simulink model "EREV_1_Model_RL"  (R2025a)
settings: Solver=ode4  StartTime=0.0  StopTime=2474  FixedStep=0.05  MaxStep=0.01  RelTol=1e-3
values from neighbouring files (symbols this model uses):
  Af = 2.95    [EREV_RL_Parameters.m]
  bsfc_map = [ ... (first row only)    [EREV_RL_Parameters.m]
  Cd = 0.33    [EREV_RL_Parameters.m]
  eff_map_F = [ ... (first row only)    [EREV_RL_Parameters.m]
  eff_map_R = [ ... (first row only)    [EREV_RL_Parameters.m]
  eff_spd_F_rpm = [0    1000  2000  3000  4000  5000  6000  7000  8000  9000  10000 11000 12000]    [EREV_RL_Parameters.m]
  eff_spd_R_rpm = [0    1000  2000  3000  4000  5000  6000  7000  8000  9000  10000 11000 12000 13000 14000 15000]    [EREV_RL_Parameters.m]
  eff_trq_F = [0   26   53   79   106  132  158  185  211  238  264]    [EREV_RL_Parameters.m]
  eff_trq_R = [0   30   61   91   122  152  182  213  243  274  304]    [EREV_RL_Parameters.m]
  eng_speed_bsfc = [1000  1500  2000  2500  3000  3500  4000  4500  5000]    [EREV_RL_Parameters.m]
  eng_speed_rpm = [1000  1500  2000  2500  3000  3500  4000  4500  5000  5500  6000]    [EREV_RL_Parameters.m]
  eng_sweet_spot_speed = 2200    [EREV_RL_Parameters.m]
  eng_sweet_spot_torque = 180    [EREV_RL_Parameters.m]
  eng_torque_bsfc = [0  50  100  150  200  250]    [EREV_RL_Parameters.m]
  eng_torque_curve = [180   240   265   265   255   240   220   195   170   145   120]    [EREV_RL_Parameters.m]
  f_roll = 0.008    [EREV_RL_Parameters.m]
  g = 9.81    [EREV_RL_Parameters.m]
  G_final_F = 8.0    (= 8)    [EREV_RL_Parameters.m]
  G_final_R_1st = G_1st    (= 12)    [EREV_RL_Parameters.m]
  G_final_R_2nd = G_2nd    (= 7)    [EREV_RL_Parameters.m]
  h = 0.65    [EREV_RL_Parameters.m]
  M_veh = 2165    [EREV_RL_Parameters.m]
  Q_bat_Ah = 38.3    [EREV_RL_Parameters.m]
  Q_bat_kWh = 13.8    [EREV_RL_Parameters.m]
  R_int_base = 0.15    [EREV_RL_Parameters.m]
  R_multiplier = [3.0  2.0  1.5  1.2  1.1  1.0  1.0  1.1  1.2  1.8  2.5]    [EREV_RL_Parameters.m]
  r_tire = 0.369    [EREV_RL_Parameters.m]
  rho = 1.225    [EREV_RL_Parameters.m]
  shift_duration = 0.3    [EREV_RL_Parameters.m]
  SOC_init = 0.5    [EREV_RL_Parameters.m]
  SOC_R_table = [0.0  0.1  0.2  0.3  0.4  0.5  0.6  0.7  0.8  0.9  1.0]    [EREV_RL_Parameters.m]
  T_motor_F_curve = [264  264  264   264   264   250   230   210   195   180   168                      156  145   135   126   118   111   104    98    92    87    82    77    73    68]    [EREV_RL_Parameters.m]
  T_motor_R_curve = [304  304  304   304   304   304   295   280   265   250   235                      220  205   192   180   169   159   150   141   133   126   119                      113  107   101    96    91    86    82    78    74]    [EREV_RL_Parameters.m]
  T_motor_R_max = 304    [EREV_RL_Parameters.m]
  T_wheel_brake_max = 5000    [EREV_RL_Parameters.m]
  tau_m_F = 0.02    [EREV_RL_Parameters.m]
  tau_m_R = 0.02    [EREV_RL_Parameters.m]
  theta = 0    [EREV_RL_Parameters.m]
  torque_split_F_4wd = 0.4    [EREV_RL_Parameters.m]
  torque_split_R_4wd = 0.6    [EREV_RL_Parameters.m]
  V_downshift_kph = 30    [EREV_RL_Parameters.m]
  v_regen_min = 8    [EREV_RL_Parameters.m]
  V_upshift_kph = 35    [EREV_RL_Parameters.m]
  VOC_map = No_cell * VOC_cell    [EREV_RL_Parameters.m]
  VOC_SOC = [0    0.05  0.1   0.2   0.3   0.4   0.5   0.6   0.7   0.8   0.9   0.95  1.0]    [EREV_RL_Parameters.m]
  Vt_init = 374.4    [EREV_RL_Parameters.m]
  w_motor_F_rpm = [0    500  1000  1500  2000  2500  3000  3500  4000  4500  5000                    5500  6000  6500  7000  7500  8000  8500  9000  9500  10000 10500 11000 11500 12000]    [EREV_RL_Parameters.m]
  w_motor_R_rpm = [0    500  1000  1500  2000  2500  3000  3500  4000  4500  5000                    5500  6000  6500  7000  7500  8000  8500  9000  9500  10000 10500                   11000 11500 12000 12500 13000 13500 14000 14500 15000]    [EREV_RL_Parameters.m]
undefined symbols (not defined in the file or in its folder): T_brake_max, T_wheel_max_current
libraries: simulink x2, autolibshared x1, slpidlib x1, rllib x1
(part 1 of 2)
settings Model: SimulationMode=accelerator  Creator=wnsgu  LastModifiedBy=wnsgu
settings SolverCC: ZeroCrossAlgorithm=Adaptive
settings DataIOCC: DSMLogging=off  ReturnWorkspaceOutputs=off

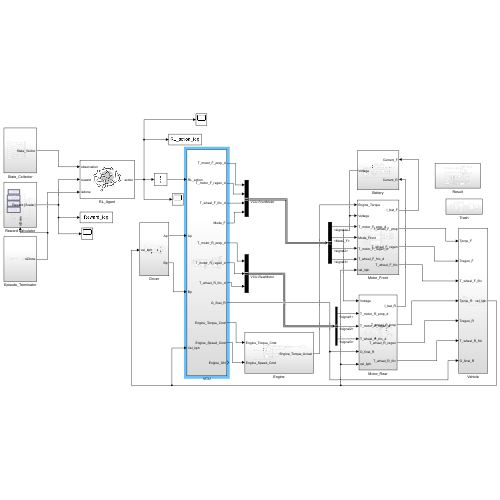
[thumbnail: Simulink's stored preview of the top-level diagram]
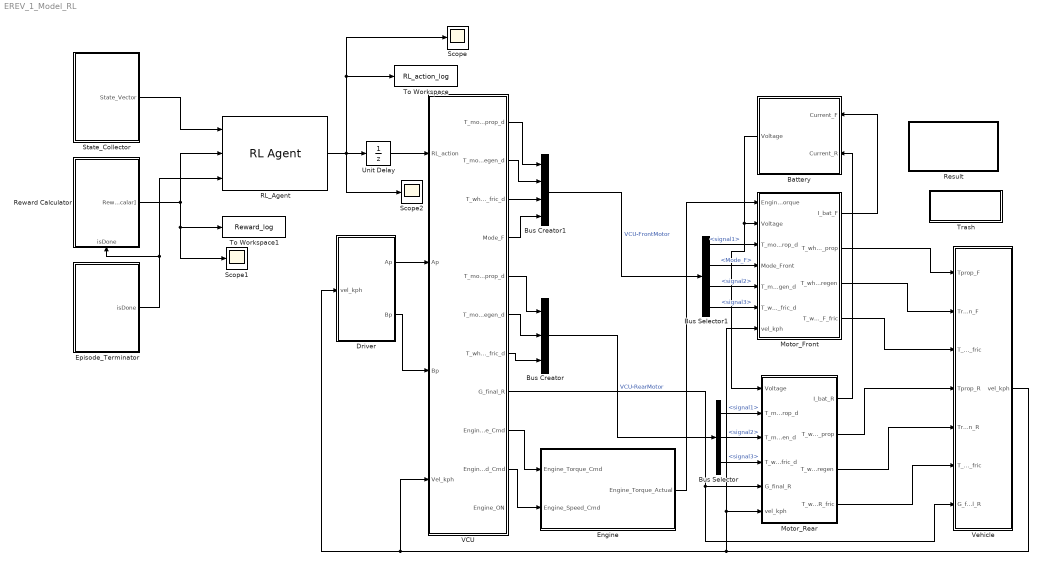
== system EREV_1_Model_RL ==
  Battery : Subsystem
      settings: PortSchema="{\"entries\":[{\"content\":{\"sides\":[{\"content\":{},\"type\":\"ConnectorPlacement.EquallySpacedRectSide\",\"uuid\":\"439f0e77-8416-4342-b481-750735cf5ce5\"},{\"content\":{\"side\":\"RIGHT\"},\"type\":\"ConnectorPlacement.EquallySpacedRectSide\",\"uuid\":\"9523e7eb-47b9-4e0c-8038-141b83390da7\"},{\"content\":{\"connectorIds\":[\"In1\",\"In2\"],\"side\":\"TOP\"},\"type\":\"ConnectorPlacement.EquallySpacedRectSide\",\"uuid\":\"5c1be694-faa9-41f0-8cd7-b694ba64a7e5\"},{\"content\":{\"connectorIds\":[\"Out1\"],\"side\":\"BOTTOM\"},\"type\":\"ConnectorPlacement.EquallySpacedRectSide\",\"uuid\":\"71711254-1c62-4381-9e1d-0f8c6cd96e13\"}]},\"type\":\"ConnectorPlacement.EquallySpacedConnector\",\"uuid\":\"675be46a-f4a3-46ab-8639-2a4821ad0461\"}],\"packageUris\":[\"http://schema.mathworks.com/mf0/Connector/R2020b\"],\"version\":\"1.0\"}"
  Bus Creator : BusCreator  Inputs=3
  Bus Creator1 : BusCreator  Inputs=4
  Bus Selector : BusSelector  OutputSignals=signal1,signal2,signal3
  Bus Selector1 : BusSelector  OutputSignals=signal1,Mode_F,signal2,signal3
  Driver : Subsystem
  Engine : Subsystem
      settings: PortSchema="{\"entries\":[{\"content\":{\"sides\":[{\"content\":{\"connectorIds\":[\"Out1\"]},\"type\":\"ConnectorPlacement.EquallySpacedRectSide\",\"uuid\":\"b19a6c52-e995-4cc1-a102-0e3cd4878d2e\"},{\"content\":{\"connectorIds\":[\"In1\",\"In2\"],\"side\":\"RIGHT\"},\"type\":\"ConnectorPlacement.EquallySpacedRectSide\",\"uuid\":\"94e23d2a-046b-4832-bf19-f0caf19abac1\"},{\"content\":{\"side\":\"TOP\"},\"type\":\"ConnectorPlacement.EquallySpacedRectSide\",\"uuid\":\"5633464f-1f19-4555-82ba-daafa5aadce4\"}]},\"type\":\"ConnectorPlacement.EquallySpacedConnector\",\"uuid\":\"3cf45f49-ebfb-4ab6-bab2-429e9c87361e\"}],\"packageUris\":[\"http://schema.mathworks.com/mf0/Connector/R2020b\"],\"version\":\"1.0\"}"
  Episode_Terminator : Subsystem
  Motor_Front : Subsystem
  Motor_Rear : Subsystem
  RL_Agent : rllib/RL Agent  Agent=agent  ExternalActionAsInput=off  ProvideLastAction=off  ProvideCumRwd=off  TreatAsDirectFeedthrough=on  UseStrictObservationDataTypes=off
  Result : Subsystem
  Reward Calculator : Subsystem
      settings: PortSchema="{\"entries\":[{\"content\":{\"sides\":[{\"content\":{},\"type\":\"ConnectorPlacement.EquallySpacedRectSide\",\"uuid\":\"cfaed86a-057d-4c04-868d-776f7886e6b3\"},{\"content\":{\"connectorIds\":[\"Out1\"],\"side\":\"RIGHT\"},\"type\":\"ConnectorPlacement.EquallySpacedRectSide\",\"uuid\":\"d11a40b4-e160-4fac-ae26-3ae90e992ab0\"},{\"content\":{\"side\":\"TOP\"},\"type\":\"ConnectorPlacement.EquallySpacedRectSide\",\"uuid\":\"52ab05fd-eff5-43dc-9a3c-d65837210fcf\"},{\"content\":{\"connectorIds\":[\"In1\"],\"side\":\"BOTTOM\"},\"type\":\"ConnectorPlacement.EquallySpacedRectSide\",\"uuid\":\"e3afb124-135f-4d45-89ab-9c20129580e4\"}]},\"type\":\"ConnectorPlacement.EquallySpacedConnector\",\"uuid\":\"1111a298-f3ef-4593-8227-a04b6f8dfe1f\"}],\"packageUris\":[\"http://schema.mathworks.com/mf0/Connector/R2020b\"],\"version\":\"1.0\"}"
  Scope : Scope
      settings: ActiveDisplayYMinimum=1  ActiveDisplayYMaximum=3  DataLoggingVariableName=ScopeData20
  Scope1 : Scope
      settings: ActiveDisplayYMinimum=-0.0074059355050510745  ActiveDisplayYMaximum=0.0037360945819499259  DataLoggingVariableName=ScopeData19
  Scope2 : Scope
      settings: ActiveDisplayYMinimum=-1  ActiveDisplayYMaximum=1  DataLoggingVariableName=ScopeData2
  State_Collector : Subsystem
  To Workspace : ToWorkspace  VariableName=RL_action_log  SaveFormat=Timeseries  SampleTime=-1
  To Workspace1 : ToWorkspace  VariableName=Reward_log  SaveFormat=Timeseries  SampleTime=-1
  Trash : Subsystem
  Unit Delay : UnitDelay  SampleTime=-1  HasFrameUpgradeWarning=on
  VCU : Subsystem
  Vehicle : Subsystem
  wires:
  Driver/2(Bp) -> VCU/3(Bp)
  Vehicle/1(vel_kph) -> VCU/4(Vel_kph), Driver/1(vel_kph), Motor_Rear/6(vel_kph), Motor_Front/7(vel_kph)
  Driver/1(Ap) -> VCU/2(Ap)
  VCU/9(Engine_Torque_Cmd) -> Engine/2(Engine_Torque_Cmd)
  VCU/10(Engine_Speed_Cmd) -> Engine/1(Engine_Speed_Cmd)
  Engine/1(Engine_Torque_Actual) -> Motor_Front/1(Engine_Torque)
  Motor_Front/2(T_wheel_F_prop) -> Vehicle/1(Tprop_F)
  Motor_Front/3(T_wheel_F_regen) -> Vehicle/2(Tregen_F)
  Motor_Front/4(T_wheel_F_fric) -> Vehicle/3(T_wheel_F_fric)
  Battery/1(Voltage) -> Motor_Rear/1(Voltage), Motor_Front/2(Voltage)
  Motor_Rear/1(I_bat_R) -> Battery/2(Current_R)
  Motor_Front/1(I_bat_F) -> Battery/1(Current_F)
  Motor_Rear/2(T_wheel_R_prop) -> Vehicle/4(Tprop_R)
  Motor_Rear/3(T_wheel_R_regen) -> Vehicle/5(Tregen_R)
  Motor_Rear/4(T_wheel_R_fric) -> Vehicle/6(T_wheel_R_fric)
  VCU/8(G_final_R) -> Motor_Rear/5(G_final_R), Vehicle/7(G_final_R)
  VCU/5(T_motor_R_prop_d) -> Bus Creator/1
  VCU/6(T_motor_R_regen_d) -> Bus Creator/2
  VCU/7(T_wheel_R_fric_d) -> Bus Creator/3
  Bus Creator/1 -> Bus Selector/1  "VCU-RearMotor"
  Bus Selector/2 -> Motor_Rear/3(T_motor_R_regen_d)  "<signal2>"
  Bus Selector/1 -> Motor_Rear/2(T_motor_R_prop_d)  "<signal1>"
  Bus Selector/3 -> Motor_Rear/4(T_wheel_R_fric_d)  "<signal3>"
  VCU/4(Mode_F) -> Bus Creator1/4
  Bus Creator1/1 -> Bus Selector1/1  "VCU-FrontMotor"
  VCU/1(T_motor_F_prop_d) -> Bus Creator1/1
  VCU/2(T_motor_F_regen_d) -> Bus Creator1/2
  VCU/3(T_wheel_F_fric_d) -> Bus Creator1/3
  Bus Selector1/1 -> Motor_Front/3(T_motor_F_prop_d)  "<signal1>"
  Bus Selector1/4 -> Motor_Front/6(T_wheel_F_fric_d)  "<signal3>"
  Reward Calculator/1(Reward [Scalar]) -> RL_Agent/2, Scope1/1, To Workspace1/1
  RL_Agent/1 -> Scope/1, To Workspace/1, Scope2/1, Unit Delay/1
  State_Collector/1(State_Vector) -> RL_Agent/1
  Episode_Terminator/1(isDone) -> RL_Agent/3, Reward Calculator/1(isDone)
  Bus Selector1/2 -> Motor_Front/4(Mode_Front)  "<Mode_F>"
  Bus Selector1/3 -> Motor_Front/5(T_motor_F_regen_d)  "<signal2>"
  Unit Delay/1 -> VCU/1(RL_action)

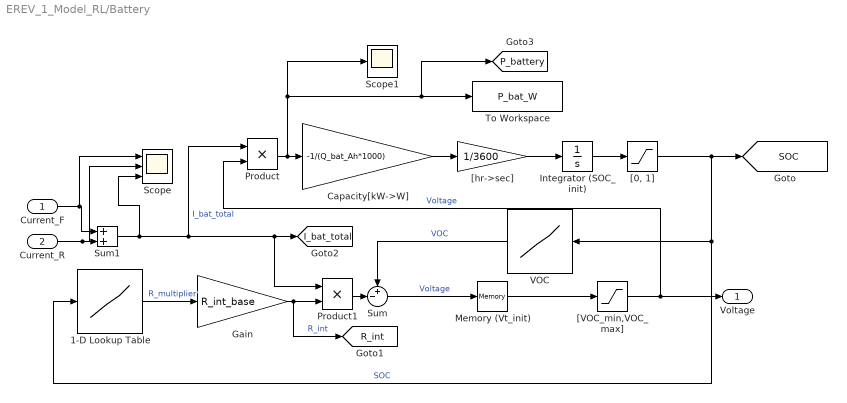
== system EREV_1_Model_RL/Battery ==
  Current_F : Inport
  Current_R : Inport  Port=2
  1-D Lookup Table : Lookup_n-D  NumberOfTableDimensions=1  BreakpointsForDimension1=SOC_R_table  Table=R_multiplier  InternalRulePriority=Speed  RndMeth=Simplest
  Capacity[kW->W] : Gain  Gain=-1/(Q_bat_Ah*1000)
  Gain : Gain  Gain=R_int_base
  Integrator (SOC_init) : Integrator  InitialCondition=SOC_init
  Memory (Vt_init) : Memory  InitialCondition=Vt_init
  Product : Product
  Product1 : Product
  Scope : Scope  NumInputPorts=3
      settings: ActiveDisplayYMinimum=-1  ActiveDisplayYMaximum=1  DataLoggingVariableName=ScopeData4
  Scope1 : Scope
      settings: ActiveDisplayYMinimum=-1  ActiveDisplayYMaximum=1  DataLoggingVariableName=ScopeData9
  Sum : Sum  Inputs=+-|
  Sum1 : Sum
  To Workspace : ToWorkspace  VariableName=P_bat_W  SaveFormat=Timeseries  SampleTime=-1
  VOC : Lookup_n-D  NumberOfTableDimensions=1  BreakpointsForDimension1=VOC_SOC  Table=VOC_map  InternalRulePriority=Speed  RndMeth=Simplest
  "[0, 1]" : Saturate  UpperLimit=1  LowerLimit=0
  "[VOC_min,VOC_max]" : Saturate  UpperLimit=max(VOC_map)  LowerLimit=min(VOC_map)
  "[hr->sec]" : Gain  Gain=1/3600
  Voltage : Outport
  tag scope: I_bat_total=global, P_battery=global, R_int=global, SOC=global
  wires:
  "[VOC_min,VOC_max]"/1 -> Product/2, Voltage/1  "Voltage"
  Product1/1 -> Sum/2
  Sum/1 -> Memory (Vt_init)/1  "Voltage"
  Integrator (SOC_init)/1 -> "[0, 1]"/1
  "[0, 1]"/1 -> VOC/1, 1-D Lookup Table/1, [SOC]  "SOC"
  Capacity[kW->W]/1 -> "[hr->sec]"/1
  Memory (Vt_init)/1 -> "[VOC_min,VOC_max]"/1
  VOC/1 -> Sum/1  "VOC"
  "[hr->sec]"/1 -> Integrator (SOC_init)/1
  Product/1 -> Scope1/1, [P_battery], To Workspace/1, Capacity[kW->W]/1
  Sum1/1 -> Scope/3, [I_bat_total], Product1/1, Product/1  "I_bat_total"
  Current_R/1 -> Scope/2, Sum1/2
  Current_F/1 -> Scope/1, Sum1/1
  1-D Lookup Table/1 -> Gain/1  "R_multiplier"
  Gain/1 -> Product1/2, [R_int]  "R_int"

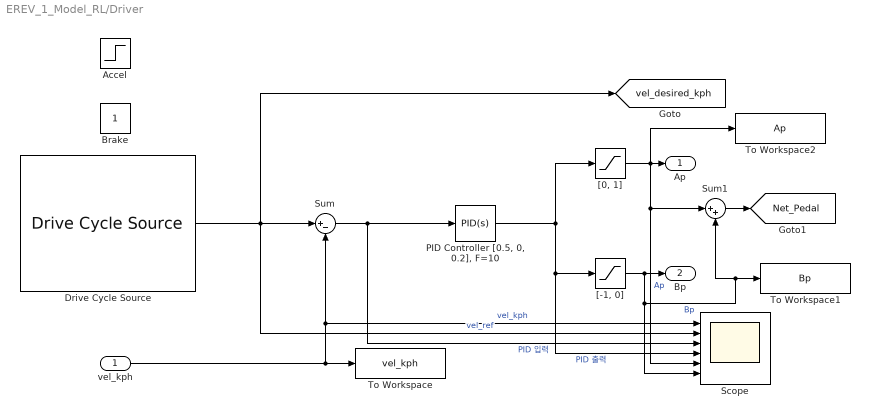
== system EREV_1_Model_RL/Driver ==
  vel_kph : Inport
  Accel : Step  SampleTime=0
  Brake : Constant
  Drive Cycle Source : autolibshared/Drive Cycle Source  cycleVar=FTP75  fileVar=cycleFTP75.mat  tfinal="2474  seconds, Cyclic"  cycleRepeat=on  outAccPort=off  outGearPort=off  gearList=No gear data  t_wot1=5  xdot_woto=0  xdot_wot1=30  t_wot2=20  xdot_wot2=0  t_wotend=30  srcUnit=m/s  outUnit=km/h  srcAccUnit=m/s/s  outAccUnit=m/s^2  dt=0  aMode=1  faultOption=off  velBnd=2  velBndUnit=mph  inUnit=m/s  timeBnd=1  failOption=off  stopSim=off  maxFaultCnt=10  maxFaultTime=2  maxTotFaultTime=15  traceOption=off  dtTrace=1  traceWindow=10  lastDCname=FTP75  lastOutUnit=mph  lastDT=0  lastTB=1  lastSB=2  forceCalcBound=off
  "PID Controller [0.5, 0, 0.2], F=10" : slpidlib/PID Controller  Controller=PID  Form=Parallel  TimeDomain=Continuous-time  UseExternalTs=off  SampleTime=-1  IntegratorMethod=Forward Euler  FilterMethod=Forward Euler  ControllerParametersSource=internal  P=0.5  I=0  UseKiTs=off  D=0.2  UseExternalDerivativeSource=off  N=10  UseFilter=on  TunerSelectOption=Transfer Function Based (PID Tuner App)  InitialConditionSource=internal  InitialConditionForIntegrator=0  InitialConditionForFilter=0  DifferentiatorICPrevScaledInput=0  ExternalReset=none  TrackingMode=off  Kt=1  LimitOutput=off  SatLimitsSource=internal  UpperSaturationLimit=inf  LowerSaturationLimit=-inf  LinearizeAsGain=on  AntiWindupMode=none  Kb=1  LimitIntegrator=off  UpperIntegratorSaturationLimit=inf  LowerIntegratorSaturationLimit=-inf  POutMin=[]  POutMax=[]  IOutMin=[]  IOutMax=[]  DOutMin=[]  DOutMax=[]  NOutMin=[]  NOutMax=[]  SumOutMin=[]  SumOutMax=[]  SaturationOutMin=[]  SaturationOutMax=[]  PParamMin=[]  PParamMax=[]  IParamMin=[]  IParamMax=[]  DParamMin=[]  DParamMax=[]  NParamMin=[]  NParamMax=[]  KbParamMin=[]  KbParamMax=[]  KtParamMin=[]  KtParamMax=[]  KbOutMin=[]  KbOutMax=[]  KtOutMin=[]  KtOutMax=[]  IntegratorOutMin=[]  IntegratorOutMax=[]  FilterOutMin=[]  FilterOutMax=[]  SumI1OutMin=[]  SumI1OutMax=[]  SumI2OutMin=[]  SumI2OutMax=[]  SumI3OutMin=[]  SumI3OutMax=[]  SumI4OutMin=[]  SumI4OutMax=[]  SumDOutMin=[]  SumDOutMax=[]  DifferentiatorOutMin=[]  DifferentiatorOutMax=[]  FilterDiffOutCoefMin=[]  FilterDiffOutCoefMax=[]  ReciprocalOutMin=[]  ReciprocalOutMax=[]  SumDenOutMin=[]  SumDenOutMax=[]  SumNumOutMin=[]  SumNumOutMax=[]  DivideOutMin=[]  DivideOutMax=[]  UdiffTsProdOutMin=[]  UdiffTsProdOutMax=[]  NTsProdOutMin=[]  NTsProdOutMax=[]  UintegralTsProdOutMin=[]  UintegralTsProdOutMax=[]  UngainTsProdOutMin=[]  UngainTsProdOutMax=[]  ClampingZeroOutDataTypeStr=Inherit: Inherit via back propagation  ClampingZeroOutMin=[]  ClampingZeroOutMax=[]  FilterDenConstantOutDataTypeStr=Inherit: Inherit via back propagation  FilterDenConstantOutMin=[]  FilterDenConstantOutMax=[]  PCopyOutDataTypeStr=Inherit: Inherit via back propagation  PCopyOutMin=[]  PCopyOutMax=[]  NCopyOutDataTypeStr=Inherit: Inherit via back propagation  NCopyOutMin=[]  NCopyOutMax=[]  IntegratorContinuousStateAttributes=''  IntegratorStateMustResolveToSignalObject=off  IntegratorRTWStateStorageClass=Auto  FilterContinuousStateAttributes=''  FilterStateMustResolveToSignalObject=off  FilterRTWStateStorageClass=Auto  ParallelPVariant=InternalParameters  IdealPVariant=Disabled  IVariant=InternalParameters  DVariant=InternalParameters  IntegratorVariant=Continuous  SatVariant=Disabled  AWVariant=Passthrough  PCopyVariant=Disabled  TRVariant=Disabled  FdbkBlocksVariant=Forward  IdealPFdbkVariant=Disabled  SatFdbkVariant=Disabled  DerivativeFilterVariant=ContFilter  NVariant=InternalParameters  NCopyVariant=Disabled  FilterICVariant=InternalICsFilter  IntegratorICVariant=InternalICs  ExternalResetVariant=Disabled  TRSumVariant=Passthrough  SumFdbkVariant=Disabled  SumVariant=Sum_PID  TsampFilterVariant=InternalTs  TsampNgainVariant=Passthrough  TsampIntegralVariant=Disabled_SignalSpec  ExternalSaturationOutDataTypeStr=Inherit: Same as second input  DerivativeSourceVariant=ErrorSignal  PreIntVariant=InternalPreInt
  Scope : Scope  NumInputPorts=6
      settings: ActiveDisplayYMinimum=-73.935455172202552  ActiveDisplayYMaximum=154.10393946357803  DataLoggingVariableName=ScopeData11
  Sum : Sum  Inputs=|+-
  Sum1 : Sum  Inputs=|++
  To Workspace : ToWorkspace  VariableName=vel_kph  SaveFormat=Timeseries  SampleTime=-1
  To Workspace1 : ToWorkspace  VariableName=Bp  SaveFormat=Timeseries  SampleTime=-1
  To Workspace2 : ToWorkspace  VariableName=Ap  SaveFormat=Timeseries  SampleTime=-1
  "[-1, 0]" : Saturate  UpperLimit=0  LowerLimit=-1
  "[0, 1]" : Saturate  UpperLimit=1  LowerLimit=0
  Ap : Outport
  Bp : Outport  Port=2
  tag scope: Net_Pedal=global, vel_desired_kph=global
  wires:
  Drive Cycle Source/1 -> Scope/2, [vel_desired_kph], Sum/1  "vel_ref"
  "[-1, 0]"/1 -> Sum1/2, To Workspace1/1, Scope/6, Bp/1  "Bp"
  "PID Controller [0.5, 0, 0.2], F=10"/1 -> Scope/4, "[-1, 0]"/1, "[0, 1]"/1  "PID 출력"
  vel_kph/1 -> To Workspace/1, Sum/2, Scope/1  "vel_kph"
  Sum/1 -> Scope/3, "PID Controller [0.5, 0, 0.2], F=10"/1  "PID 입력"
  "[0, 1]"/1 -> To Workspace2/1, Scope/5, Sum1/1, Ap/1  "Ap"
  Sum1/1 -> [Net_Pedal]

== system EREV_1_Model_RL/Engine ==
  Engine_Speed_Cmd : Inport
  Engine_Torque_Cmd : Inport  Port=2
  Gain : Gain  Gain=pi/30
  Gain1 : Gain  Gain=1/3600
  Min : MinMax  Inputs=2
  Product : Product
  Product1 : Product
  "Rate Limiter [Rising Slew Rate : 100]" : RateLimiter  RisingSlewLimit=100  SampleTimeMode=inherited
  Torque Max Curve : Lookup_n-D  NumberOfTableDimensions=1  BreakpointsForDimension1=eng_speed_rpm  Table=eng_torque_curve  InternalRulePriority=Speed  RndMeth=Simplest
  "[W] -> [kW]" : Gain  Gain=1/1000
  bsfc_map : Lookup_n-D  BreakpointsForDimension1=eng_speed_bsfc  BreakpointsForDimension2=eng_torque_bsfc  Table=bsfc_map  InternalRulePriority=Speed  RndMeth=Simplest
      settings: InputPortMap=u0,u1
  Engine_Torque_Actual : Outport
  tag scope: Fuel_Consumption=global
  wires:
  Engine_Speed_Cmd/1 -> Gain/1, bsfc_map/1, Torque Max Curve/1
  Engine_Torque_Cmd/1 -> Min/2
  Torque Max Curve/1 -> Min/1  "Max Torque"
  Min/1 -> "Rate Limiter [Rising Slew Rate : 100]"/1, Product1/2, bsfc_map/2  "Actual Torque"
  Gain/1 -> Product1/1  "Speed [rad/s]"
  Gain1/1 -> [Fuel_Consumption]  "Fuel_Consumption"
  Product1/1 -> "[W] -> [kW]"/1  "Power [W]"
  Product/1 -> Gain1/1
  "[W] -> [kW]"/1 -> Product/1  "Power [kW]"
  bsfc_map/1 -> Product/2  "BSFC Value [g/hr/kW]"
  "Rate Limiter [Rising Slew Rate : 100]"/1 -> Engine_Torque_Actual/1

== system EREV_1_Model_RL/Episode_Terminator ==
  Abs : Abs  SaturateOnIntegerOverflow=off
  Compare To Constant : simulink/Logic and Bit Operations/Compare To Constant  relop=>  const=10  OutDataTypeStr=boolean
  Compare To Constant1 : simulink/Logic and Bit Operations/Compare To Constant  relop=>=  const=5  OutDataTypeStr=boolean
  Data Type Conversion : DataTypeConversion  OutDataTypeStr=double  SaturateOnIntegerOverflow=off  RndMeth=Floor
  Integrator : Integrator  ExternalReset=rising  LimitOutput=on  UpperSaturationLimit=10  LowerSaturationLimit=0
  NOT : Logic  Operator=NOT  IconShape=distinctive  AllPortsSameDT=off  OutDataTypeStr=boolean
  Sum1 : Sum  Inputs=|+-
  isDone : Outport
  wires:
  Compare To Constant1/1 -> isDone/1
  Sum1/1 -> Abs/1
  [vel_kph] -> Sum1/2
  [vel_desired_kph] -> Sum1/1
  Abs/1 -> Compare To Constant/1
  Compare To Constant/1 -> Data Type Conversion/1
  Integrator/1 -> Compare To Constant1/1
  NOT/1 -> Integrator/2
  Data Type Conversion/1 -> NOT/1, Integrator/1

== system EREV_1_Model_RL/Motor_Front ==
  Engine_Torque : Inport
  Voltage : Inport  Port=2
  T_motor_F_prop_d : Inport  Port=3
  Mode_Front : Inport  Port=4
  T_motor_F_regen_d : Inport  Port=5
  T_wheel_F_fric_d : Inport  Port=6
  vel_kph : Inport  Port=7
  Demux : Demux
  Disconnect : Subsystem
  Generator : Subsystem
  Motor : Subsystem
  Multiport Switch : MultiPortSwitch  DataPortOrder=Zero-based contiguous  zeroidx=on  SaturateOnIntegerOverflow=off  InputSameDT=off
  I_bat_F : Outport
  T_wheel_F_prop : Outport  Port=2
  T_wheel_F_regen : Outport  Port=3
  T_wheel_F_fric : Outport  Port=4
  wires:
  Demux/1 -> T_wheel_F_prop/1
  Demux/2 -> T_wheel_F_regen/1
  Demux/3 -> T_wheel_F_fric/1
  Demux/4 -> I_bat_F/1
  Multiport Switch/1 -> Demux/1
  Engine_Torque/1 -> Generator/2(Engine_Torque)
  T_motor_F_prop_d/1 -> Motor/1(T_motor_F_prop_d)
  T_motor_F_regen_d/1 -> Motor/2(T_motor_F_regen_d)
  Voltage/1 -> Motor/4(Voltage), Generator/1(Voltage)
  Mode_Front/1 -> Multiport Switch/1
  Disconnect/1(Disconnect) -> Multiport Switch/2  "2WD"
  Motor/1("Motor ") -> Multiport Switch/3  "4WD"
  Generator/1(Generator) -> Multiport Switch/4  "Generation"
  vel_kph/1 -> Motor/5(vel_kph)
  T_wheel_F_fric_d/1 -> Motor/3(T_wheel_F_fric_d)

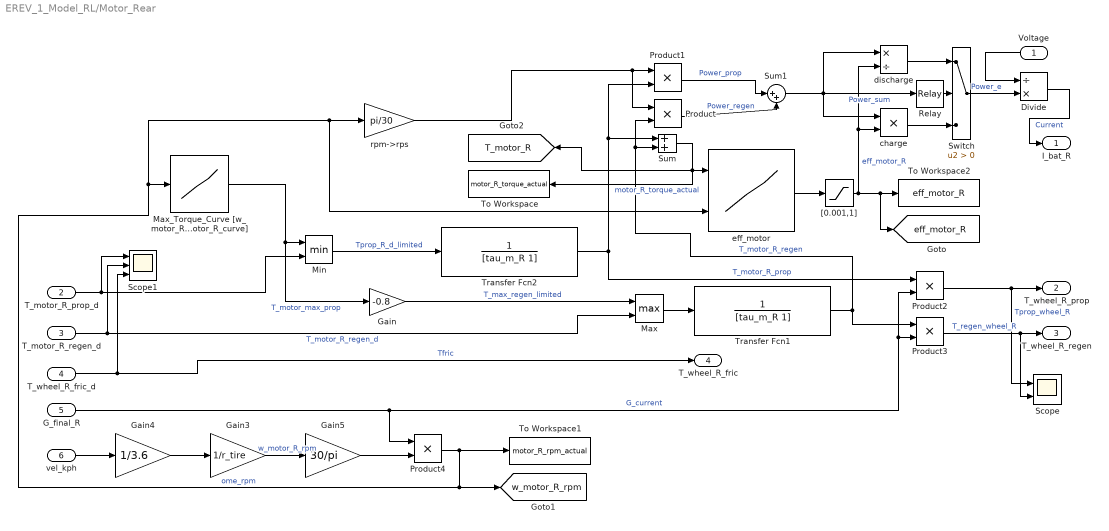
== system EREV_1_Model_RL/Motor_Rear ==
  Voltage : Inport
  T_motor_R_prop_d : Inport  Port=2
  T_motor_R_regen_d : Inport  Port=3
  T_wheel_R_fric_d : Inport  Port=4
  G_final_R : Inport  Port=5
  vel_kph : Inport  Port=6
  Divide : Product  Inputs=/*
  Gain : Gain  Gain=-0.8
  Gain3 : Gain  Gain=1/r_tire
  Gain4 : Gain  Gain=1/3.6
  Gain5 : Gain  Gain=30/pi
  Max : MinMax  Function=max  Inputs=2
  Max_Torque_Curve [w_motor_R_rpm,T_motor_R_curve] : Lookup_n-D  NumberOfTableDimensions=1  BreakpointsForDimension1=w_motor_R_rpm  Table=T_motor_R_curve  InternalRulePriority=Speed  RndMeth=Simplest
  Min : MinMax  Inputs=2
  Product{,1..4} (5 alike) : Product
  Relay : Relay  OnSwitchValue=10  OffSwitchValue=-10
  Scope : Scope  NumInputPorts=2
      settings: ActiveDisplayYMinimum=-1  ActiveDisplayYMaximum=1  DataLoggingVariableName=ScopeData5
  Scope1 : Scope  NumInputPorts=3
      settings: ActiveDisplayYMinimum=-1  ActiveDisplayYMaximum=1  DataLoggingVariableName=ScopeData6
  Sum : Sum
  Sum1 : Sum  Inputs=|++
  Switch : Switch  Criteria=u2 > Threshold  SaturateOnIntegerOverflow=off  InputSameDT=off
  To Workspace : ToWorkspace  VariableName=motor_R_torque_actual  SaveFormat=Timeseries  SampleTime=-1
  To Workspace1 : ToWorkspace  VariableName=motor_R_rpm_actual  SaveFormat=Timeseries  SampleTime=-1
  To Workspace2 : ToWorkspace  VariableName=eff_motor_R  SaveFormat=Timeseries  SampleTime=-1
  Transfer Fcn1 : TransferFcn  Denominator=[tau_m_R 1]
  Transfer Fcn2 : TransferFcn  Denominator=[tau_m_R 1]
  "[0.001,1]" : Saturate  UpperLimit=1  LowerLimit=0.001
  charge : Product
  discharge : Product  Inputs=*/
  eff_motor : Lookup_n-D  BreakpointsForDimension1=eff_trq_R  BreakpointsForDimension2=eff_spd_R_rpm  Table=eff_map_R*0.01  InternalRulePriority=Speed  RndMeth=Simplest
      settings: InputPortMap=u0,u1
  rpm->rps : Gain  Gain=pi/30
  I_bat_R : Outport
  T_wheel_R_prop : Outport  Port=2
  T_wheel_R_regen : Outport  Port=3
  T_wheel_R_fric : Outport  Port=4
  tag scope: T_motor_R=global, eff_motor_R=global, w_motor_R_rpm=global
  wires:
  discharge/1 -> Switch/1
  Product4/1 -> eff_motor/2, rpm->rps/1, Max_Torque_Curve [w_motor_R_rpm,T_motor_R_curve]/1, [w_motor_R_rpm], To Workspace1/1  "ome_rpm"
  "[0.001,1]"/1 -> [eff_motor_R], To Workspace2/1, discharge/2, charge/2  "eff_motor_R"
  Switch/1 -> Divide/2  "Power_e"
  rpm->rps/1 -> Product/1, Product1/1
  Voltage/1 -> Divide/1
  Sum1/1 -> Relay/1, discharge/1, charge/1  "Power_sum"
  Divide/1 -> I_bat_R/1  "Current"
  charge/1 -> Switch/3
  eff_motor/1 -> "[0.001,1]"/1
  Product/1 -> Sum1/2  "Power_regen"
  Product1/1 -> Sum1/1  "Power_prop"
  Sum/1 -> eff_motor/1, [T_motor_R], To Workspace/1  "motor_R_torque_actual"
  Relay/1 -> Switch/2
  Min/1 -> Transfer Fcn2/1  "Tprop_R_d_limited"
  Transfer Fcn2/1 -> Product2/1, Sum/1, Product1/2  "T_motor_R_prop"
  Max_Torque_Curve [w_motor_R_rpm,T_motor_R_curve]/1 -> Min/1, Gain/1  "T_motor_max_prop"
  T_motor_R_prop_d/1 -> Scope1/1, Min/2
  Gain/1 -> Max/1  "T_max_regen_limited"
  T_motor_R_regen_d/1 -> Max/2, Scope1/2  "T_motor_R_regen_d"
  Max/1 -> Transfer Fcn1/1
  Transfer Fcn1/1 -> Product3/1, Sum/2, Product/2  "T_motor_R_regen"
  G_final_R/1 -> Product2/2, Product3/2, Product4/1  "G_current"
  Product2/1 -> Scope/1, T_wheel_R_prop/1  "Tprop_wheel_R"
  Product3/1 -> Scope/2, T_wheel_R_regen/1  "T_regen_wheel_R"
  vel_kph/1 -> Gain4/1
  Gain4/1 -> Gain3/1
  Gain3/1 -> Gain5/1  "w_motor_R_rpm"
  Gain5/1 -> Product4/2
  T_wheel_R_fric_d/1 -> Scope1/3, T_wheel_R_fric/1  "Tfric"

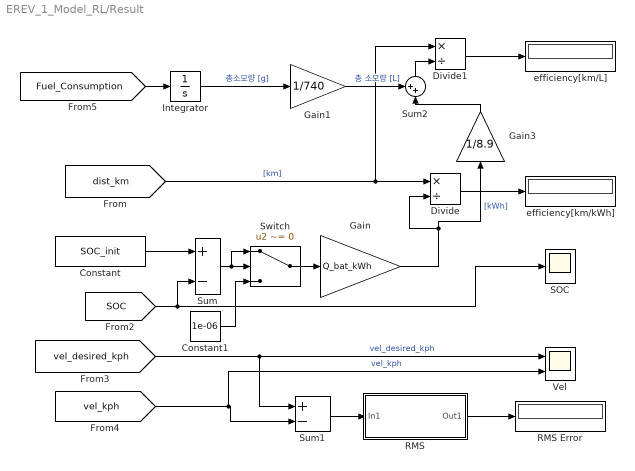
== system EREV_1_Model_RL/Result ==
  Constant : Constant  Value=SOC_init
  Constant1 : Constant  Value=1e-06
  Divide : Product  Inputs=*/
  Divide1 : Product  Inputs=*/
  Gain : Gain  Gain=Q_bat_kWh
  Gain1 : Gain  Gain=1/740
  Gain3 : Gain  Gain=1/8.9
  Integrator : Integrator
  RMS : Subsystem
  RMS Error : Display
  SOC : Scope
      settings: ActiveDisplayYMinimum=0.45615237264927222  ActiveDisplayYMaximum=0.89462864615655024
  Sum : Sum  Inputs=+-
  Sum1 : Sum  Inputs=+-
  Sum2 : Sum  Inputs=++|
  Switch : Switch  Criteria=u2 ~= 0  SaturateOnIntegerOverflow=off  InputSameDT=off
  Vel : Scope  NumInputPorts=2
      settings: ActiveDisplayYMinimum=-8.8916034999999969  ActiveDisplayYMaximum=80.024431499999992
  efficiency[km/L] : Display
  efficiency[km/kWh] : Display
  wires:
  [vel_desired_kph] -> Sum1/1, Vel/1  "vel_desired_kph"
  [vel_kph] -> Vel/2, Sum1/2  "vel_kph"
  Sum1/1 -> RMS/1(In1)
  Constant/1 -> Sum/1
  RMS/1(Out1) -> RMS Error/1
  [SOC] -> SOC/1, Sum/2
  Switch/1 -> Gain/1
  Sum/1 -> Switch/1, Switch/2
  Constant1/1 -> Switch/3
  Gain/1 -> Gain3/1, Divide/2  "[kWh]"
  Divide1/1 -> efficiency[km/L]/1
  [dist_km] -> Divide/1, Divide1/1  "[km]"
  Integrator/1 -> Gain1/1  "총소모량 [g]"
  Gain1/1 -> Sum2/1  "총 소모량 [L]"
  Sum2/1 -> Divide1/2
  [Fuel_Consumption] -> Integrator/1
  Divide/1 -> efficiency[km/kWh]/1
  Gain3/1 -> Sum2/2

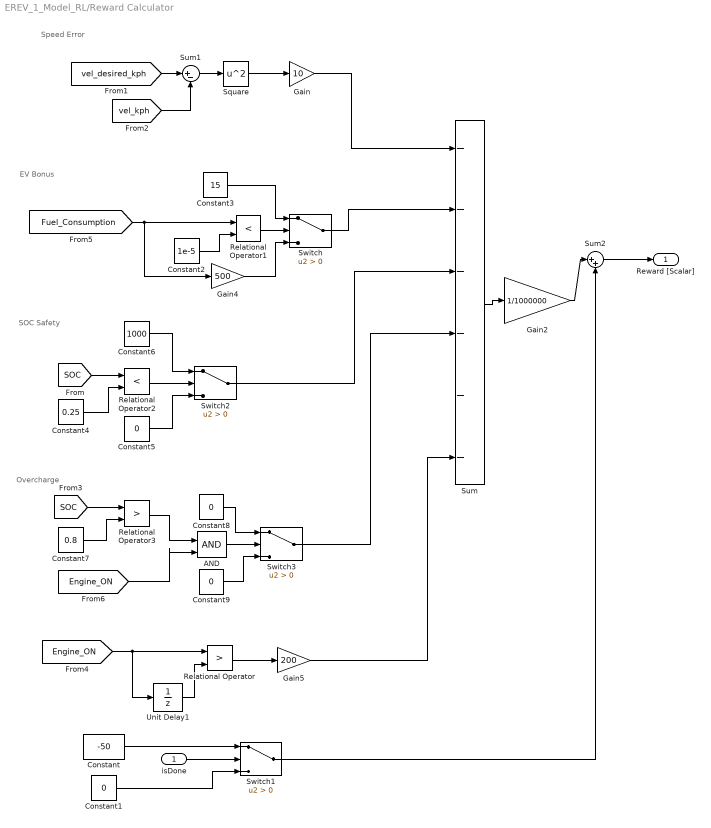
== system EREV_1_Model_RL/Reward Calculator ==
  note: Overcharge
  note: SOC Safety
  note: EV Bonus
  note: Speed Error
  isDone : Inport
  AND : Logic  IconShape=distinctive  AllPortsSameDT=off  OutDataTypeStr=boolean
  Constant : Constant  Value=-50
  Constant{1,5,8..9} (4 alike) : Constant  Value=0
  Constant2 : Constant  Value=1e-5
  Constant3 : Constant  Value=15
  Constant4 : Constant  Value=0.25
  Constant6 : Constant  Value=1000
  Constant7 : Constant  Value=0.8
  Gain : Gain  Gain=10
  Gain2 : Gain  Gain=1/1000000
  Gain4 : Gain  Gain=500
  Gain5 : Gain  Gain=200
  Relational Operator : RelationalOperator  Operator=>  OutDataTypeStr=boolean  RndMeth=Simplest  InputSameDT=off
  Relational Operator1 : RelationalOperator  Operator=<  OutDataTypeStr=boolean  RndMeth=Simplest  InputSameDT=off
  Relational Operator2 : RelationalOperator  Operator=<  OutDataTypeStr=boolean  RndMeth=Simplest  InputSameDT=off
  Relational Operator3 : RelationalOperator  Operator=>  OutDataTypeStr=boolean  RndMeth=Simplest  InputSameDT=off
  Square : Math  Operator=square
  Sum : Sum  Inputs=------
  Sum1 : Sum  Inputs=|+-
  Sum2 : Sum  Inputs=|++
  Switch{,1..3} (4 alike) : Switch  Criteria=u2 > Threshold  SaturateOnIntegerOverflow=off  InputSameDT=off
  Unit Delay1 : UnitDelay  SampleTime=-1  HasFrameUpgradeWarning=on
  Reward [Scalar] : Outport
  wires:
  [vel_desired_kph] -> Sum1/1
  [vel_kph] -> Sum1/2
  Sum1/1 -> Square/1
  isDone/1 -> Switch1/2
  Constant/1 -> Switch1/1
  Constant1/1 -> Switch1/3
  Square/1 -> Gain/1
  Gain/1 -> Sum/1
  Sum/1 -> Gain2/1
  Sum2/1 -> Reward [Scalar]/1
  Gain2/1 -> Sum2/1
  Switch1/1 -> Sum2/2
  [Engine_ON] -> Relational Operator/1, Unit Delay1/1
  Unit Delay1/1 -> Relational Operator/2
  Relational Operator/1 -> Gain5/1
  Gain5/1 -> Sum/6
  [Fuel_Consumption] -> Gain4/1, Relational Operator1/1
  Constant2/1 -> Relational Operator1/2
  Relational Operator1/1 -> Switch/2
  Gain4/1 -> Switch/3
  Constant3/1 -> Switch/1
  [SOC] -> Relational Operator2/1
  Constant4/1 -> Relational Operator2/2
  Relational Operator2/1 -> Switch2/2
  Constant6/1 -> Switch2/1
  Constant5/1 -> Switch2/3
  Switch/1 -> Sum/2
  Switch2/1 -> Sum/3
  [SOC] -> Relational Operator3/1
  Constant7/1 -> Relational Operator3/2
  Relational Operator3/1 -> AND/1
  [Engine_ON] -> AND/2
  AND/1 -> Switch3/2
  Constant8/1 -> Switch3/1
  Constant9/1 -> Switch3/3
  Switch3/1 -> Sum/4

== system EREV_1_Model_RL/State_Collector ==
  Integrator : Integrator
  Mux : Mux  Inputs=8
  Product : Product
  Unit Delay1 : UnitDelay  SampleTime=-1  HasFrameUpgradeWarning=on
  단위변환 : Subsystem
  State_Vector : Outport
  wires:
  [vel_kph] -> Integrator/1, Mux/1  "vel_kph [km/h]"
  Integrator/1 -> Mux/2  "accel [m/s^2]"
  [Net_Pedal] -> Mux/3  "Ap+Bp [-1, 1]"
  [SOC] -> Mux/4  "SOC [0, 1]"
  [Gear_R] -> Unit Delay1/1  "Gear_R [1, 2]"
  [eff_motor_R] -> Mux/6  "eff_motor_R"
  Product/1 -> Mux/7  "Power_demand [kW]"
  Mux/1 -> State_Vector/1
  Unit Delay1/1 -> Mux/5
  [w_motor_R_rpm] -> 단위변환/1(rpm)
  단위변환/1(rad/s) -> Product/2
  [T_motor_R] -> Product/1
  [vel_desired_kph] -> Mux/8  "vel_desired_kph [km/h]"

== system EREV_1_Model_RL/Trash ==
  Engine_Command_Gen : Subsystem  Commented=on
  Engine_ONOFF_Logic : Subsystem  Commented=on
  Front_Rear_Distribution : Subsystem  Commented=on
  Gear_Ratio_Selection : Subsystem  Commented=on
  Gear_Selection : Subsystem  Commented=on
  Mode_Selection : Subsystem  Commented=on
  Motor_Limit_Check : Subsystem  Commented=on
  Output_Saturation : Subsystem  Commented=on
  Pedal_to_Wheel_Torque : Subsystem  Commented=on
  RegenFriction_Distribution : Subsystem  Commented=on
  RegenFriction_Distribution1 : Subsystem  Commented=on
  SOC_Monitoring : Subsystem  Commented=on
  Wheel_to_Motor_Torque : Subsystem  Commented=on
  Wheel_to_Motor_Torque1 : Subsystem  Commented=on
  wires:
  SOC_Monitoring/1(sys_mode) -> Mode_Selection/1(sys_mode)

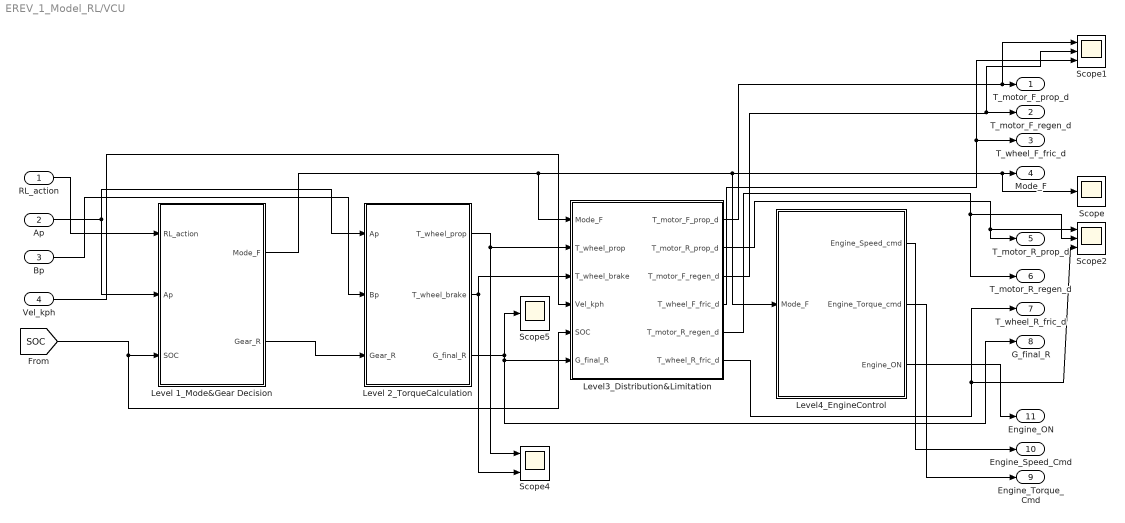
== system EREV_1_Model_RL/VCU ==
  RL_action : Inport
  Ap : Inport  Port=2
  Bp : Inport  Port=3
  Vel_kph : Inport  Port=4
  Level 1_Mode&Gear Decision : Subsystem
  Level 2_TorqueCalculation : Subsystem
  Level3_Distribution&Limitation : Subsystem
  Level4_EngineControl : Subsystem
  Scope : Scope
      settings: ActiveDisplayYMinimum=-1  ActiveDisplayYMaximum=1  DataLoggingVariableName=ScopeData2
  Scope1 : Scope  NumInputPorts=3
      settings: ActiveDisplayYMinimum=-1  ActiveDisplayYMaximum=1  DataLoggingVariableName=ScopeData7
  Scope2 : Scope  NumInputPorts=3
      settings: ActiveDisplayYMinimum=-1  ActiveDisplayYMaximum=1  DataLoggingVariableName=ScopeData8
  Scope4 : Scope  NumInputPorts=2
      settings: ActiveDisplayYMinimum=-164.78073168707266  ActiveDisplayYMaximum=197.13547955305179  DataLoggingVariableName=ScopeData10
  Scope5 : Scope
      settings: ActiveDisplayYMinimum=-1.4999999999999996  ActiveDisplayYMaximum=13.5  DataLoggingVariableName=ScopeData18
  T_motor_F_prop_d : Outport
  T_motor_F_regen_d : Outport  Port=2
  T_wheel_F_fric_d : Outport  Port=3
  Mode_F : Outport  Port=4
  T_motor_R_prop_d : Outport  Port=5
  T_motor_R_regen_d : Outport  Port=6
  T_wheel_R_fric_d : Outport  Port=7
  G_final_R : Outport  Port=8
  Engine_Torque_Cmd : Outport  Port=9
  Engine_Speed_Cmd : Outport  Port=10
  Engine_ON : Outport  Port=11
  wires:
  Vel_kph/1 -> Level3_Distribution&Limitation/4(Vel_kph)
  Ap/1 -> Level 2_TorqueCalculation/1(Ap), Level 1_Mode&Gear Decision/2(Ap)
  Bp/1 -> Level 2_TorqueCalculation/2(Bp)
  [SOC] -> Level3_Distribution&Limitation/5(SOC), Level 1_Mode&Gear Decision/3(SOC)
  Level 1_Mode&Gear Decision/1(Mode_F) -> Level4_EngineControl/1(Mode_F), Mode_F/1, Scope/1, Level3_Distribution&Limitation/1(Mode_F)
  Level 2_TorqueCalculation/1(T_wheel_prop) -> Scope4/1, Level3_Distribution&Limitation/2(T_wheel_prop)
  Level 2_TorqueCalculation/2(T_wheel_brake) -> Level3_Distribution&Limitation/3(T_wheel_brake), Scope4/2
  Level 2_TorqueCalculation/3(G_final_R) -> Level3_Distribution&Limitation/6(G_final_R), G_final_R/1, Scope5/1
  Level4_EngineControl/2(Engine_Torque_cmd) -> Engine_Torque_Cmd/1
  Level4_EngineControl/1(Engine_Speed_cmd) -> Engine_Speed_Cmd/1
  Level3_Distribution&Limitation/1(T_motor_F_prop_d) -> Scope1/1, T_motor_F_prop_d/1
  Level3_Distribution&Limitation/3(T_motor_F_regen_d) -> Scope1/2, T_motor_F_regen_d/1
  Level3_Distribution&Limitation/4(T_wheel_F_fric_d) -> Scope1/3, T_wheel_F_fric_d/1
  Level3_Distribution&Limitation/6(T_wheel_R_fric_d) -> T_wheel_R_fric_d/1, Scope2/3
  Level3_Distribution&Limitation/2(T_motor_R_prop_d) -> T_motor_R_prop_d/1, Scope2/1
  Level3_Distribution&Limitation/5(T_motor_R_regen_d) -> T_motor_R_regen_d/1, Scope2/2
  RL_action/1 -> Level 1_Mode&Gear Decision/1(RL_action)
  Level 1_Mode&Gear Decision/2(Gear_R) -> Level 2_TorqueCalculation/3(Gear_R)
  Level4_EngineControl/3(Engine_ON) -> Engine_ON/1

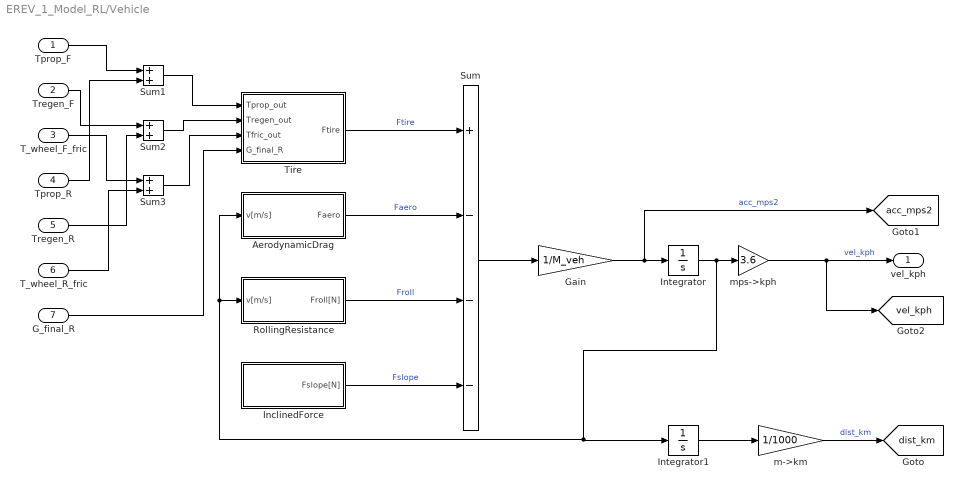
== system EREV_1_Model_RL/Vehicle ==
  Tprop_F : Inport
  Tregen_F : Inport  Port=2
  T_wheel_F_fric : Inport  Port=3
  Tprop_R : Inport  Port=4
  Tregen_R : Inport  Port=5
  T_wheel_R_fric : Inport  Port=6
  G_final_R : Inport  Port=7
  AerodynamicDrag : Subsystem
  Gain : Gain  Gain=1/M_veh
  InclinedForce : Subsystem
  Integrator : Integrator
  Integrator1 : Integrator
  RollingResistance : Subsystem
  Sum : Sum  Inputs=+---
  Sum1 : Sum
  Sum2 : Sum
  Sum3 : Sum
  Tire : Subsystem
  m->km : Gain  Gain=1/1000
  mps->kph : Gain  Gain=3.6
  vel_kph : Outport
  tag scope: acc_mps2=global, dist_km=global, vel_kph=global
  wires:
  Gain/1 -> Integrator/1, [acc_mps2]  "acc_mps2"
  Tire/1(Ftire) -> Sum/1  "Ftire"
  Sum/1 -> Gain/1
  Integrator/1 -> AerodynamicDrag/1(v[m/s]), RollingResistance/1(v[m/s]), Integrator1/1, mps->kph/1
  AerodynamicDrag/1(Faero) -> Sum/2  "Faero"
  m->km/1 -> [dist_km]  "dist_km"
  RollingResistance/1(Froll[N]) -> Sum/3  "Froll"
  mps->kph/1 -> [vel_kph], vel_kph/1  "vel_kph"
  InclinedForce/1(Fslope[N]) -> Sum/4  "Fslope"
  Integrator1/1 -> m->km/1
  Sum2/1 -> Tire/2(Tregen_out)
  Sum1/1 -> Tire/1(Tprop_out)
  Sum3/1 -> Tire/3(Tfric_out)
  T_wheel_R_fric/1 -> Sum3/2
  T_wheel_F_fric/1 -> Sum3/1
  Tregen_R/1 -> Sum2/2
  Tprop_R/1 -> Sum1/2
  Tprop_F/1 -> Sum1/1
  Tregen_F/1 -> Sum2/1
  G_final_R/1 -> Tire/4(G_final_R)

== system EREV_1_Model_RL/Motor_Front/Disconnect ==
  Constant : Constant  Value=0
  Mux : Mux
  Disconnect : Outport
  wires:
  Mux/1 -> Disconnect/1
  Constant/1 -> Mux/1, Mux/4, Mux/3, Mux/2

== system EREV_1_Model_RL/Motor_Front/Generator ==
  Voltage : Inport
  Engine_Torque : Inport  Port=2
  Constant : Constant  Value=0
  Divide1 : Product  Inputs=*/
  EngineSpeed[rpm] : Constant  Value=eng_sweet_spot_speed
  Gain1 : Gain  Gain=pi/30
  Mux : Mux
  Product2 : Product
  발전효율 : Gain  Gain=-0.92
  Generator : Outport
  wires:
  Mux/1 -> Generator/1
  Constant/1 -> Mux/1, Mux/2, Mux/3
  EngineSpeed[rpm]/1 -> Gain1/1
  Gain1/1 -> Product2/2  "w_gen"
  Engine_Torque/1 -> Product2/1
  Product2/1 -> 발전효율/1  "P_mech"
  발전효율/1 -> Divide1/1
  Voltage/1 -> Divide1/2
  Divide1/1 -> Mux/4

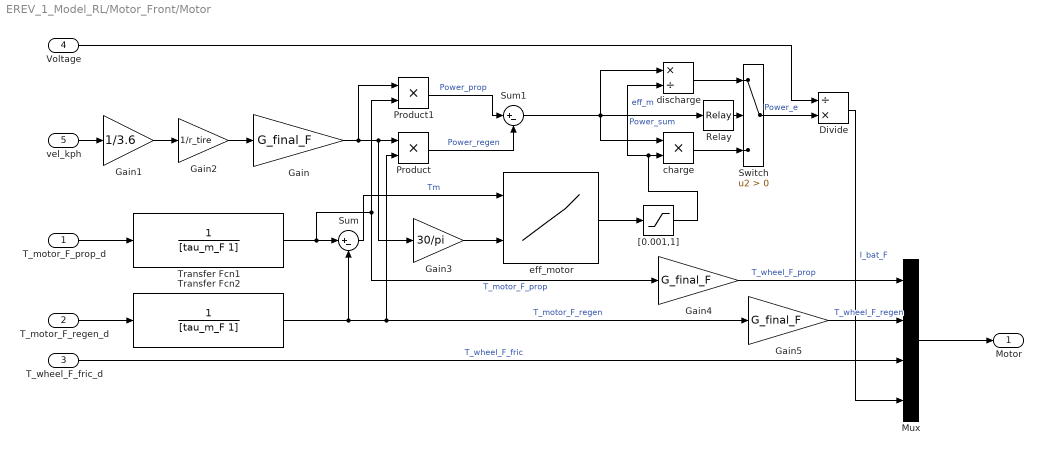
== system EREV_1_Model_RL/Motor_Front/Motor ==
  T_motor_F_prop_d : Inport
  T_motor_F_regen_d : Inport  Port=2
  T_wheel_F_fric_d : Inport  Port=3
  Voltage : Inport  Port=4
  vel_kph : Inport  Port=5
  Divide : Product  Inputs=/*
  Gain : Gain  Gain=G_final_F
  Gain1 : Gain  Gain=1/3.6
  Gain2 : Gain  Gain=1/r_tire
  Gain3 : Gain  Gain=30/pi
  Gain4 : Gain  Gain=G_final_F
  Gain5 : Gain  Gain=G_final_F
  Mux : Mux
  Product : Product
  Product1 : Product
  Relay : Relay  OnSwitchValue=10  OffSwitchValue=-10
  Sum : Sum  Inputs=|+-
  Sum1 : Sum  Inputs=|+-
  Switch : Switch  Criteria=u2 > Threshold  SaturateOnIntegerOverflow=off  InputSameDT=off
  Transfer Fcn1 : TransferFcn  Denominator=[tau_m_F 1]
  Transfer Fcn2 : TransferFcn  Denominator=[tau_m_F 1]
  "[0.001,1]" : Saturate  UpperLimit=1  LowerLimit=0.001
  charge : Product
  discharge : Product  Inputs=*/
  eff_motor : Lookup_n-D  BreakpointsForDimension1=eff_trq_F  BreakpointsForDimension2=eff_spd_F_rpm  Table=eff_map_F*0.01  InternalRulePriority=Speed  RndMeth=Simplest
      settings: InputPortMap=u0,u1
  "Motor " : Outport
  wires:
  T_motor_F_regen_d/1 -> Transfer Fcn2/1
  Divide/1 -> Mux/4  "I_bat_F"
  Product/1 -> Sum1/2  "Power_regen"
  Switch/1 -> Divide/2  "Power_e"
  Product1/1 -> Sum1/1  "Power_prop"
  Voltage/1 -> Divide/1
  Sum1/1 -> Relay/1, discharge/1, charge/1  "Power_sum"
  Sum/1 -> eff_motor/1  "Tm"
  T_wheel_F_fric_d/1 -> Mux/3  "T_wheel_F_fric"
  Transfer Fcn2/1 -> Gain5/1, Product/2, Sum/2  "T_motor_F_regen"
  Transfer Fcn1/1 -> Sum/1, Gain4/1, Product1/2  "T_motor_F_prop"
  charge/1 -> Switch/3
  discharge/1 -> Switch/1
  Relay/1 -> Switch/2
  T_motor_F_prop_d/1 -> Transfer Fcn1/1
  "[0.001,1]"/1 -> discharge/2, charge/2  "eff_m"
  Gain/1 -> Gain3/1, Product/1, Product1/1
  eff_motor/1 -> "[0.001,1]"/1
  Mux/1 -> "Motor "/1
  vel_kph/1 -> Gain1/1
  Gain1/1 -> Gain2/1
  Gain2/1 -> Gain/1
  Gain3/1 -> eff_motor/2
  Gain5/1 -> Mux/2  "T_wheel_F_regen"
  Gain4/1 -> Mux/1  "T_wheel_F_prop"

== system EREV_1_Model_RL/Result/RMS ==
  In1 : Inport
  Clock : Clock
  Constant : Constant  Value=1e-9
  Divide : Product  Inputs=*/
  Integrator : Integrator
  Root : Sqrt
  Square : Math  Operator=square
  Switch : Switch  Criteria=u2 > Threshold  SaturateOnIntegerOverflow=off  InputSameDT=off
  To Workspace : ToWorkspace  VariableName=sim_time  SaveFormat=Timeseries  SampleTime=-1
  time step : Gain  Gain=0.01
  Out1 : Outport
  wires:
  In1/1 -> Square/1
  Square/1 -> time step/1
  time step/1 -> Integrator/1
  Integrator/1 -> Divide/1
  Root/1 -> Out1/1
  Divide/1 -> Root/1
  Constant/1 -> Switch/3
  Clock/1 -> To Workspace/1, Switch/2, Switch/1  "t_out"
  Switch/1 -> Divide/2

== system EREV_1_Model_RL/State_Collector/단위변환 ==
  rpm : Inport
  Gain : Gain  Gain=2*pi/60
  Gain1 : Gain  Gain=1/1000
  rad/s : Outport
  wires:
  rpm/1 -> Gain/1
  Gain1/1 -> rad/s/1
  Gain/1 -> Gain1/1

== system EREV_1_Model_RL/Trash/Engine_Command_Gen ==
  Engine_ON : Inport
  MATLAB Function : MATLAB Function  TreatAsAtomicUnit=on
  Engine_Speed_cmd : Outport
  Engine_Torque_cmd : Outport  Port=2
  wires:
  Engine_ON/1 -> MATLAB Function/1(Engien_ON)
  MATLAB Function/1(Engine_Speed_cmd) -> Engine_Speed_cmd/1
  MATLAB Function/2(Engine_Torque_cmd) -> Engine_Torque_cmd/1

== system EREV_1_Model_RL/Trash/Engine_ONOFF_Logic ==
  Mode_F : Inport
  Constant : Constant  Value=2
  Equal : RelationalOperator  Operator===  OutDataTypeStr=boolean  RndMeth=Simplest  InputSameDT=off
  Engine_ON : Outport
  wires:
  Mode_F/1 -> Equal/1
  Constant/1 -> Equal/2
  Equal/1 -> Engine_ON/1

== system EREV_1_Model_RL/Trash/Front_Rear_Distribution ==
  Tprop_motor_d : Inport
  Mode_F : Inport  Port=2
  Constant : Constant  Value=G_final_F
  MATLAB Function : MATLAB Function  TreatAsAtomicUnit=on
  Tprop_F_d : Outport
  Tprop_R_d : Outport  Port=2
  wires:
  Mode_F/1 -> MATLAB Function/2(Mode_F)
  Tprop_motor_d/1 -> MATLAB Function/1(Tprop_motor_d)
  Constant/1 -> MATLAB Function/3(G_final_R)
  MATLAB Function/1(Tprop_F_d) -> Tprop_F_d/1
  MATLAB Function/2(Tprop_R_d) -> Tprop_R_d/1

== system EREV_1_Model_RL/Trash/Gear_Ratio_Selection ==
  Gear_R : Inport
  Constant : Constant  Value=G_final_R_1st
  Constant1 : Constant  Value=G_final_R_2nd
  Switch : Switch  Criteria=u2 > Threshold  Threshold=1.5  SaturateOnIntegerOverflow=off  InputSameDT=off
  G_final_R : Outport
  wires:
  Gear_R/1 -> Switch/2
  Constant/1 -> Switch/1
  Constant1/1 -> Switch/3
  Switch/1 -> G_final_R/1

== system EREV_1_Model_RL/Trash/Gear_Selection ==
  Vel_kph : Inport
  Ap : Inport  Port=2
  MATLAB Function : MATLAB Function  TreatAsAtomicUnit=on
  Memory : Memory  InitialCondition=1
  Gear_R : Outport
  wires:
  Vel_kph/1 -> MATLAB Function/1(Vel_kph)
  Ap/1 -> MATLAB Function/2(Ap)
  MATLAB Function/1(Gear_R) -> Memory/1
  Memory/1 -> Gear_R/1

== system EREV_1_Model_RL/Trash/Mode_Selection ==
  sys_mode : Inport
  Ap : Inport  Port=2
  MATLAB Function : MATLAB Function  TreatAsAtomicUnit=on
  Mode_F : Outport
  wires:
  Ap/1 -> MATLAB Function/2(Ap)
  sys_mode/1 -> MATLAB Function/1(sys_mode)
  MATLAB Function/1(Mode_F) -> Mode_F/1

== system EREV_1_Model_RL/Trash/Motor_Limit_Check ==
  Tprop_motor_d : Inport
  MATLAB Function : MATLAB Function  TreatAsAtomicUnit=on
  Saturation : Saturate  UpperLimit=203  LowerLimit=0
  Tprop_limited : Outport
  wires:
  Tprop_motor_d/1 -> MATLAB Function/1(Tprop_motor_d)
  MATLAB Function/1(Tprop_limited) -> Saturation/1
  Saturation/1 -> Tprop_limited/1

== system EREV_1_Model_RL/Trash/Output_Saturation ==
  Tprop_R_d : Inport
  Out1 : Outport
  wires:
  Tprop_R_d/1 -> Out1/1

== system EREV_1_Model_RL/Trash/Pedal_to_Wheel_Torque ==
  Ap : Inport
  Bp : Inport  Port=2
  Gain1 : Gain  Gain=T_brake_max
  Gain2 : Gain  Gain=T_wheel_max_current
  Saturation : Saturate
  Saturation1 : Saturate
  T_wheel_prop : Outport
  T_wheel_brake : Outport  Port=2
  wires:
  Bp/1 -> Gain1/1
  Ap/1 -> Gain2/1
  Gain2/1 -> Saturation/1
  Saturation/1 -> T_wheel_prop/1
  Saturation1/1 -> T_wheel_brake/1
  Gain1/1 -> Saturation1/1

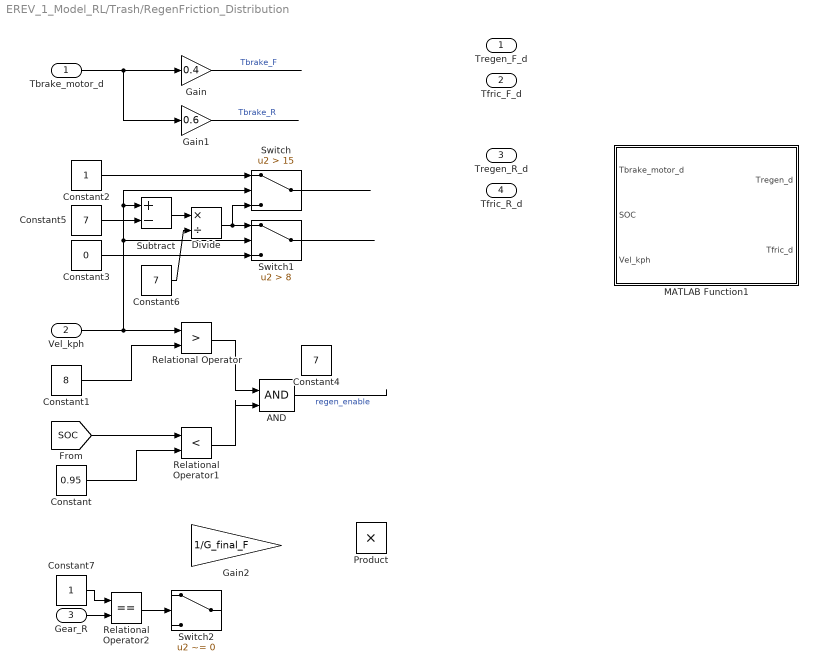
== system EREV_1_Model_RL/Trash/RegenFriction_Distribution ==
  Tbrake_motor_d : Inport
  Vel_kph : Inport  Port=2
  Gear_R : Inport  Port=3
  AND : Logic  IconShape=distinctive  AllPortsSameDT=off  OutDataTypeStr=boolean
  Constant : Constant  Value=0.95
  Constant1 : Constant  Value=8
  Constant2 : Constant
  Constant3 : Constant  Value=0
  Constant4 : Constant  Value=7
  Constant5 : Constant  Value=7
  Constant6 : Constant  Value=7
  Constant7 : Constant
  Divide : Product  Inputs=*/
  Gain : Gain  Gain=0.4
  Gain1 : Gain  Gain=0.6
  Gain2 : Gain  Gain=1/G_final_F
  MATLAB Function1 : MATLAB Function  TreatAsAtomicUnit=on
  Product : Product
  Relational Operator : RelationalOperator  Operator=>  OutDataTypeStr=boolean  RndMeth=Simplest  InputSameDT=off
  Relational Operator1 : RelationalOperator  Operator=<  OutDataTypeStr=boolean  RndMeth=Simplest  InputSameDT=off
  Relational Operator2 : RelationalOperator  Operator===  OutDataTypeStr=boolean  RndMeth=Simplest  InputSameDT=off
  Subtract : Sum  Inputs=+-
  Switch : Switch  Criteria=u2 > Threshold  Threshold=15  SaturateOnIntegerOverflow=off  InputSameDT=off
  Switch1 : Switch  Criteria=u2 > Threshold  Threshold=8  SaturateOnIntegerOverflow=off  InputSameDT=off
  Switch2 : Switch  Criteria=u2 ~= 0  SaturateOnIntegerOverflow=off  InputSameDT=off
  Tregen_F_d : Outport
  Tfric_F_d : Outport  Port=2
  Tregen_R_d : Outport  Port=3
  Tfric_R_d : Outport  Port=4
  wires:
  Tbrake_motor_d/1 -> Gain1/1, Gain/1
  ? -> Tfric_F_d/1
  ? -> Tregen_F_d/1
  Gain/1 -> ?  "Tbrake_F"
  Gain1/1 -> ?  "Tbrake_R"
  [SOC] -> Relational Operator1/1
  Constant/1 -> Relational Operator1/2
  Constant1/1 -> Relational Operator/2
  Relational Operator/1 -> AND/1
  Relational Operator1/1 -> AND/2
  AND/1 -> ?  "regen_enable"
  Constant3/1 -> Switch1/3
  Constant2/1 -> Switch/1
  Vel_kph/1 -> Subtract/1, Switch/2, Switch1/2, Relational Operator/1
  Switch/1 -> ?
  Constant5/1 -> Subtract/2
  Subtract/1 -> Divide/1
  Divide/1 -> Switch/3, Switch1/1
  Constant6/1 -> Divide/2
  Switch1/1 -> ?
  Gear_R/1 -> Relational Operator2/2
  Relational Operator2/1 -> Switch2/2
  Constant7/1 -> Relational Operator2/1

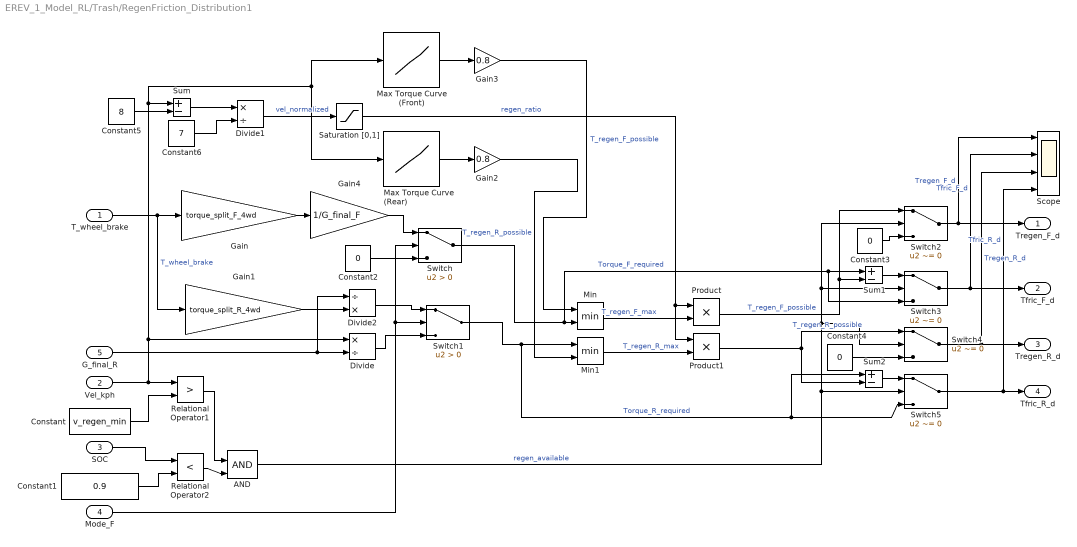
== system EREV_1_Model_RL/Trash/RegenFriction_Distribution1 ==
  T_wheel_brake : Inport
  Vel_kph : Inport  Port=2
  SOC : Inport  Port=3
  Mode_F : Inport  Port=4
  G_final_R : Inport  Port=5
  AND : Logic  IconShape=distinctive  AllPortsSameDT=off  OutDataTypeStr=boolean
  Constant : Constant  Value=v_regen_min
  Constant1 : Constant  Value=0.9
  Constant2 : Constant  Value=0
  Constant3 : Constant  Value=0
  Constant4 : Constant  Value=0
  Constant5 : Constant  Value=8
  Constant6 : Constant  Value=7
  Divide : Product  Inputs=*/
  Divide1 : Product  Inputs=*/
  Divide2 : Product  Inputs=/*
  Gain : Gain  Gain=torque_split_F_4wd
  Gain1 : Gain  Gain=torque_split_R_4wd
  Gain2 : Gain  Gain=0.8
  Gain3 : Gain  Gain=0.8
  Gain4 : Gain  Gain=1/G_final_F
  Max Torque Curve (Front) : Lookup_n-D  NumberOfTableDimensions=1  BreakpointsForDimension1=w_motor_F_rpm  Table=T_motor_F_curve  InternalRulePriority=Speed  RndMeth=Simplest
  Max Torque Curve (Rear) : Lookup_n-D  NumberOfTableDimensions=1  BreakpointsForDimension1=w_motor_R_rpm  Table=T_motor_R_curve  InternalRulePriority=Speed  RndMeth=Simplest
  Min : MinMax  Inputs=2
  Min1 : MinMax  Inputs=2
  Product : Product
  Product1 : Product
  Relational Operator1 : RelationalOperator  Operator=>  OutDataTypeStr=boolean  RndMeth=Simplest  InputSameDT=off
  Relational Operator2 : RelationalOperator  Operator=<  OutDataTypeStr=boolean  RndMeth=Simplest  InputSameDT=off
  Saturation [0,1] : Saturate  UpperLimit=1  LowerLimit=0
  Scope : Scope  NumInputPorts=4
      settings: ActiveDisplayYMinimum=-1.1158015712526246  ActiveDisplayYMaximum=10.042214141273623  DataLoggingVariableName=ScopeData12
  Sum : Sum  Inputs=+-
  Sum1 : Sum  Inputs=+-
  Sum2 : Sum  Inputs=+-
  Switch : Switch  Criteria=u2 > Threshold  SaturateOnIntegerOverflow=off  InputSameDT=off
  Switch1 : Switch  Criteria=u2 > Threshold  SaturateOnIntegerOverflow=off  InputSameDT=off
  Switch{2..5} (4 alike) : Switch  Criteria=u2 ~= 0  SaturateOnIntegerOverflow=off  InputSameDT=off
  Tregen_F_d : Outport
  Tfric_F_d : Outport  Port=2
  Tregen_R_d : Outport  Port=3
  Tfric_R_d : Outport  Port=4
  wires:
  T_wheel_brake/1 -> Gain1/1, Gain/1  "T_wheel_brake"
  Vel_kph/1 -> Divide/1, Max Torque Curve (Front)/1, Max Torque Curve (Rear)/1, Sum/1, Relational Operator1/1
  Constant/1 -> Relational Operator1/2
  SOC/1 -> Relational Operator2/1
  Relational Operator1/1 -> AND/1
  Relational Operator2/1 -> AND/2
  Mode_F/1 -> Switch/2, Switch1/2
  Constant2/1 -> Switch/3
  Switch2/1 -> Scope/1, Tregen_F_d/1  "Tregen_F_d"
  Switch3/1 -> Scope/2, Tfric_F_d/1  "Tfric_F_d"
  Switch5/1 -> Scope/4, Tfric_R_d/1  "Tfric_R_d"
  Switch4/1 -> Scope/3, Tregen_R_d/1  "Tregen_R_d"
  Constant1/1 -> Relational Operator2/2
  Constant5/1 -> Sum/2
  Constant6/1 -> Divide1/2
  Sum/1 -> Divide1/1
  Divide1/1 -> Saturation [0,1]/1  "vel_normalized"
  AND/1 -> Switch5/2, Switch2/2, Switch3/2, Switch4/2  "regen_available"
  Switch/1 -> Switch3/3, Sum1/1, Min/2  "Torque_F_required"
  Max Torque Curve (Front)/1 -> Gain3/1
  Max Torque Curve (Rear)/1 -> Gain2/1
  Saturation [0,1]/1 -> Product1/1, Product/1  "regen_ratio"
  Gain2/1 -> Min1/2  "T_regen_R_possible"
  Gain3/1 -> Min/1  "T_regen_F_possible"
  Min/1 -> Product/2  "T_regen_F_max"
  Min1/1 -> Product1/2  "T_regen_R_max"
  Product/1 -> Switch2/1, Sum1/2  "T_regen_F_possible"
  Product1/1 -> Sum2/2, Switch4/1  "T_regen_R_possible"
  Sum1/1 -> Switch3/1
  Switch1/1 -> Switch5/3, Sum2/1, Min1/1  "Torque_R_required"
  Constant3/1 -> Switch2/3
  Constant4/1 -> Switch4/3
  Sum2/1 -> Switch5/1
  Gain/1 -> Gain4/1
  Gain4/1 -> Switch/1
  G_final_R/1 -> Divide2/1, Divide/2
  Gain1/1 -> Divide2/2
  Divide/1 -> Switch1/3
  Divide2/1 -> Switch1/1

== system EREV_1_Model_RL/Trash/SOC_Monitoring ==
  SOC : Inport
  Constant : Constant  Value=2
  Constant1 : Constant  Value=0
  Memory : Memory
  Switch : Switch  Criteria=u2 > Threshold  Threshold=0.3  SaturateOnIntegerOverflow=off  InputSameDT=off
  Switch1 : Switch  Criteria=u2 > Threshold  Threshold=0.7  SaturateOnIntegerOverflow=off  InputSameDT=off
  sys_mode : Outport
  wires:
  SOC/1 -> Switch1/2, Switch/2
  Constant/1 -> Switch/3
  Constant1/1 -> Switch1/1
  Memory/1 -> Switch/1
  Switch/1 -> Switch1/3
  Switch1/1 -> Memory/1, sys_mode/1

== system EREV_1_Model_RL/Trash/Wheel_to_Motor_Torque ==
  T_wheel_prop : Inport
  T_wheel_brake : Inport  Port=2
  Gear_R : Inport  Port=3
  Divide : Product  Inputs=*/
  Divide1 : Product  Inputs=/*
  Saturation [0,203 : Saturate  UpperLimit=203  LowerLimit=0
  Saturation [0,203] : Saturate  UpperLimit=203  LowerLimit=0
  Tprop_motor_d : Outport
  Tbrake_motor_d : Outport  Port=2
  wires:
  T_wheel_brake/1 -> Divide1/2
  T_wheel_prop/1 -> Divide/1
  Gear_R/1 -> Divide1/1, Divide/2
  Divide/1 -> Saturation [0,203]/1
  Divide1/1 -> Saturation [0,203/1
  Saturation [0,203/1 -> Tbrake_motor_d/1
  Saturation [0,203]/1 -> Tprop_motor_d/1

== system EREV_1_Model_RL/Trash/Wheel_to_Motor_Torque1 ==
  T_wheel_prop : Inport
  T_wheel_brake : Inport  Port=2
  Gear_R : Inport  Port=3
  Divide : Product  Inputs=*/
  Divide1 : Product  Inputs=/*
  Saturation [-500,0] : Saturate  UpperLimit=0  LowerLimit=-500
  Saturation [0,568] : Saturate  UpperLimit=568  LowerLimit=0
  Tprop_motor_d : Outport
  Tbrake_motor_d : Outport  Port=2
  wires:
  T_wheel_brake/1 -> Divide1/2
  T_wheel_prop/1 -> Divide/1
  Gear_R/1 -> Divide1/1, Divide/2
  Divide/1 -> Saturation [0,568]/1
  Divide1/1 -> Saturation [-500,0]/1
  Saturation [-500,0]/1 -> Tbrake_motor_d/1
  Saturation [0,568]/1 -> Tprop_motor_d/1

== system EREV_1_Model_RL/VCU/Level 1_Mode&Gear Decision ==
  RL_action : Inport
  Ap : Inport  Port=2
  SOC : Inport  Port=3
  MATLAB Function : MATLAB Function  TreatAsAtomicUnit=on  SystemSampleTime=0.05
  Previous : Subsystem  Commented=on
  To Workspace : ToWorkspace  VariableName=Mode_F  SaveFormat=Timeseries  SampleTime=-1
  Mode_F : Outport
  Gear_R : Outport  Port=2
  wires:
  RL_action/1 -> MATLAB Function/1(RL_Action)
  SOC/1 -> MATLAB Function/2(SOC)
  MATLAB Function/2(Mode_F) -> To Workspace/1, Mode_F/1
  MATLAB Function/1(Target_Gear) -> Gear_R/1
  Ap/1 -> MATLAB Function/3(Ap)
